simulink model "Proportional_Integral_Control"  (R2022b)
settings: Solver=VariableStepAuto  StartTime=0.0  StopTime=100  RelTol=1e-3
settings Model: Creator=bekir  LastModifiedBy=bekir

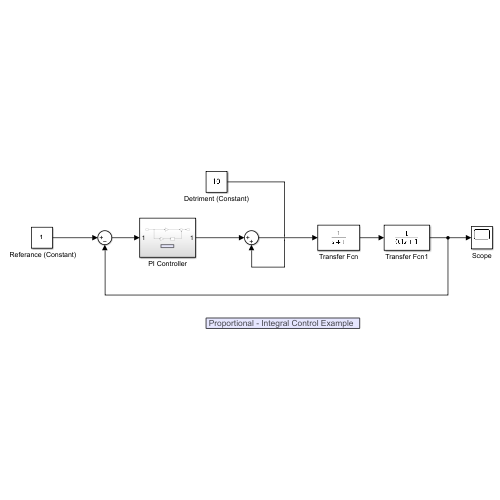
[thumbnail: Simulink's stored preview of the top-level diagram]
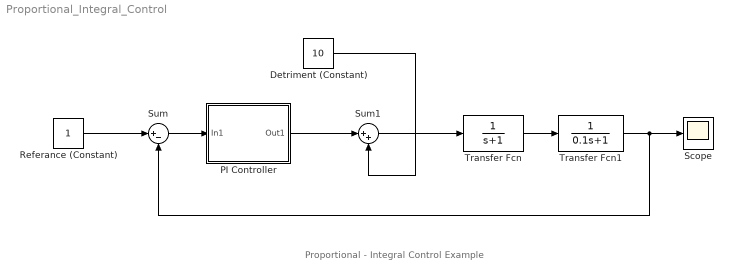
== system Proportional_Integral_Control ==
  note: Proportional - Integral Control Example
  " Referance (Constant)" : Constant
  Detriment (Constant) : Constant  Value=10
  PI Controller : Subsystem
  Scope : Scope
  Sum : Sum  Inputs=|+-
  Sum1 : Sum  Inputs=|++
  Transfer Fcn : TransferFcn  Denominator=[1 1]
  Transfer Fcn1 : TransferFcn  Denominator=[0.1 1]
  wires:
  PI Controller/1(Out1) -> Sum1/1
  " Referance (Constant)"/1 -> Sum/1
  Transfer Fcn1/1 -> Sum/2, Scope/1
  Transfer Fcn/1 -> Transfer Fcn1/1
  Sum/1 -> PI Controller/1(In1)
  Detriment (Constant)/1 -> Sum1/2
  Sum1/1 -> Transfer Fcn/1

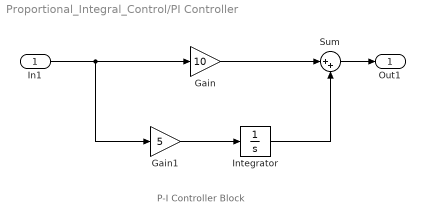
== system Proportional_Integral_Control/PI Controller ==
  note: P-I Controller Block
  In1 : Inport
  Gain : Gain  Gain=10
  Gain1 : Gain  Gain=5
  Integrator : Integrator
  Sum : Sum  Inputs=|++
  Out1 : Outport
  wires:
  In1/1 -> Gain1/1, Gain/1
  Gain1/1 -> Integrator/1
  Gain/1 -> Sum/1
  Integrator/1 -> Sum/2
  Sum/1 -> Out1/1
